simulink model "threeqiaoshiquanbo"  (R2018a)
settings: Solver=ode23tb  StartTime=0.0  StopTime=0.1  RelTol=1e-3
libraries: powerlib x16, powerlib_extras x1
settings Model: Creator=ASUS  LastModifiedBy=ASUS
settings DataIOCC: ReturnWorkspaceOutputs=on
settings DebuggingCC: UnconnectedInputMsg=none  UnconnectedOutputMsg=none  UnconnectedLineMsg=none
settings ModelReferenceCC: EnableRefExpFcnMdlSchedulingChecks=off
settings SFSimCC: SimUseLocalCustomCode=on
settings RTWCC: Description=Generic Real-Time Target  RTWUseLocalCustomCode=on

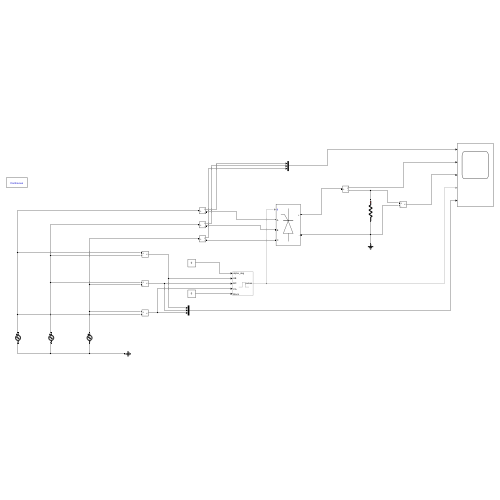
[thumbnail: Simulink's stored preview of the top-level diagram]
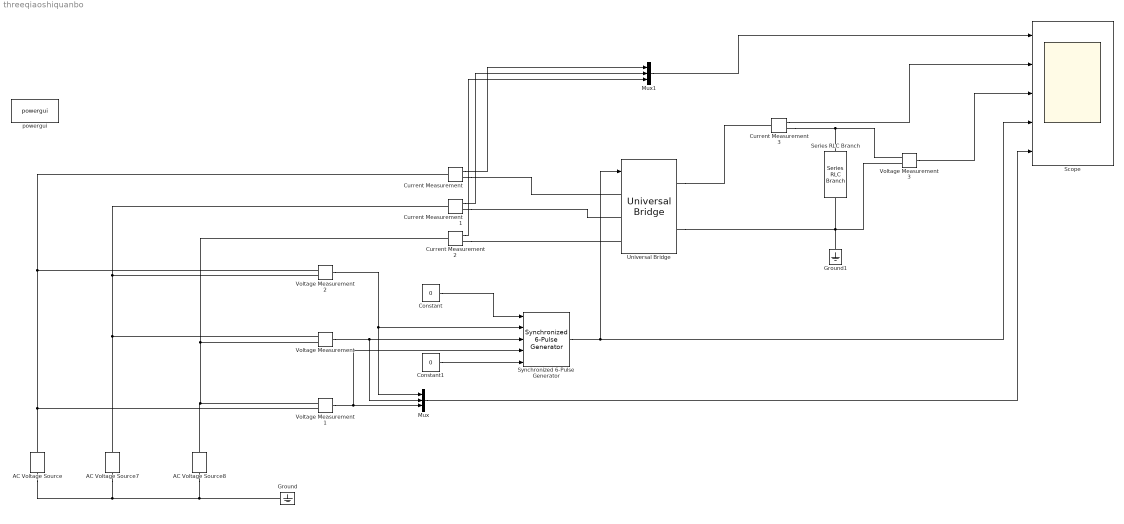
== system threeqiaoshiquanbo ==
  AC Voltage Source : powerlib/Electrical Sources/AC Voltage Source  Amplitude=380  Phase=0  Frequency=50  SampleTime=0  Measurements=None  BusType=swing  Pref=10e3  Qref=0  Qmin=-inf  Qmax=+inf
  AC Voltage Source7 : powerlib/Electrical Sources/AC Voltage Source  Amplitude=380  Phase=-120  Frequency=50  SampleTime=0  Measurements=None  BusType=swing  Pref=10e3  Qref=0  Qmin=-inf  Qmax=+inf
  AC Voltage Source8 : powerlib/Electrical Sources/AC Voltage Source  Amplitude=380  Phase=-240  Frequency=50  SampleTime=0  Measurements=None  BusType=swing  Pref=10e3  Qref=0  Qmin=-inf  Qmax=+inf
  Constant : Constant  Value=0
  Constant1 : Constant  Value=0
  Current Measurement{,1..3} (4 alike) : powerlib/Measurements/Current Measurement  PhasorSimulation=off  OutputType=Complex  PSBequivalent=0
  Ground : powerlib/Elements/Ground  LConnTagsString=a
  Ground1 : powerlib/Elements/Ground  LConnTagsString=a
  Mux : Mux  Inputs=3
  Mux1 : Mux  Inputs=3
  Scope : Scope  NumInputPorts=5
  Series RLC Branch : powerlib/Elements/Series RLC Branch  LConnTagsString=__new0  RConnTagsString=__new0  BranchType=R  Resistance=1  Inductance=0  SetiL0=off  InitialCurrent=0  Capacitance=inf  Setx0=off  InitialVoltage=0  Measurements=None
  Synchronized 6-Pulse Generator : powerlib_extras/Control  Blocks/Synchronized 6-Pulse Generator  freq=60  pwidth=10  Double_Pulse=off
  Universal Bridge : powerlib/Power Electronics/Universal Bridge  Arms=3  SnubberResistance=50  SnubberCapacitance=1e-6  Device=Thyristors  Ron=1e-3  Lon=0  ForwardVoltages="[  0  0  ]"  ForwardVoltage=0.8  GTOparameters=[ 10e-6 , 20e-6 ]  IGBTparameters=[ 1e-6 , 2e-6 ]  Measurements=All voltages and currents  Measurements_2=None  converterType=Rectifier
  Voltage Measurement{,1..3} (4 alike) : powerlib/Measurements/Voltage Measurement  PhasorSimulation=off  OutputType=Complex  PSBequivalent=0
  powergui : powerlib/powergui  Priority=1  SimulationMode=Continuous  SampleTime=50e-6  frequency=60  Iterations=50  frequencyindice=50  Pbase=100e6  ErrMax=1e-4  UnitsV=kV  UnitsW=MW  buscounter=0  FunctionMessages=off  echomessages=off  EnableUseOfTLC=off  CurrentSourceSwitches=off  DisableSnubberDevices=off  DisableRonSwitches=off  DisableVfSwitches=off  DisplayEquations=off  AutomaticDiscreteSolvers=off  SolverType=Tustin/Backward Euler (TBE)  Interpol=off  ExternalGateDelay=off  methode=off  Ts=100  x0status=blocks  SPID=on  SwTol=0  HookPort=off  NonlinearTolerance=1e-4  nMaxIteration=100  ContinueOnMaxIteration=off  RestoreLinks=warning  ResistiveCurrentMeasurement=off  Frange=[0:2:500]  Ylog=off  Xlog=on  ShowGrid=off  save=off  variable=ZData  structure=0  ZoomFFT=off  StartTime=0.0  cycles=1  DisplayStyle=1  fundamental=60  FreqAxis=off  MaxFrequency=1000  frequencyindicesteady=1  RmsSteady=1  display=off
  wires:
  Constant/1 -> Synchronized 6-Pulse Generator/1
  Voltage Measurement2/1 -> Synchronized 6-Pulse Generator/2, Mux/1
  Voltage Measurement/1 -> Synchronized 6-Pulse Generator/3, Mux/2
  Voltage Measurement1/1 -> Synchronized 6-Pulse Generator/4, Mux/3
  Constant1/1 -> Synchronized 6-Pulse Generator/5
  Synchronized 6-Pulse Generator/1 -> Scope/4, Universal Bridge/1
  Current Measurement/1 -> Mux1/1
  Current Measurement1/1 -> Mux1/2
  Current Measurement2/1 -> Mux1/3
  Mux1/1 -> Scope/1
  Current Measurement3/1 -> Scope/2
  Voltage Measurement3/1 -> Scope/3
  Mux/1 -> Scope/5
  connections:
  AC Voltage Source8/RConn1 -- Current Measurement2/LConn1 -- Voltage Measurement/LConn2 -- Voltage Measurement1/LConn1
  AC Voltage Source8/LConn1 -- AC Voltage Source/LConn1 -- AC Voltage Source7/LConn1 -- Ground/LConn1
  Voltage Measurement/LConn1 -- Current Measurement1/LConn1 -- Voltage Measurement2/LConn2 -- AC Voltage Source7/RConn1
  Voltage Measurement2/LConn1 -- Voltage Measurement1/LConn2 -- AC Voltage Source/RConn1 -- Current Measurement/LConn1
  Current Measurement2/RConn1 -- Universal Bridge/LConn3
  Current Measurement1/RConn1 -- Universal Bridge/LConn2
  Current Measurement/RConn1 -- Universal Bridge/LConn1
  Universal Bridge/RConn1 -- Current Measurement3/LConn1
  Current Measurement3/RConn1 -- Voltage Measurement3/LConn1 -- Series RLC Branch/LConn1
  Universal Bridge/RConn2 -- Ground1/LConn1 -- Voltage Measurement3/LConn2 -- Series RLC Branch/RConn1
